simulink model "svc_go_c"  (R2018a)
settings: Solver=VariableStepAuto  StartTime=0.0  StopTime=10.0  RelTol=1e-3
InitFcn:
  | svc_go_init
values from neighbouring files (symbols this model uses):
  kp = (3*Ld./N/Ts-Rs)/Lq/Iq    [est_model_paras.m]    (also in svc_go_init.m = -0.01944)
  Ld = 0.000891    [est_model_paras.m]    (also in svc_go_init.m = 0.00026)
  Ldr = 0.00026    [svc_go_init.m]
  Lq = 0.000891    [est_model_paras.m]    (also in svc_go_init.m = 0.000636)
  Lqr = 0.00053    [svc_go_init.m]
  phi_r = 0.012    [est_model_paras.m]    (also in svc_go_init.m = 0.078)
  Rs = 0.503    [est_model_paras.m]    (also in svc_go_init.m = 0.021)
  Rsr = 0.021    [svc_go_init.m]
  We = 2*pi*100    (= 628.318530718)    [est_model_paras.m]    (also in svc_go_init.m)
libraries: simulink x5
settings Model: Creator=LG-PC  LastModifiedBy=LG-PC

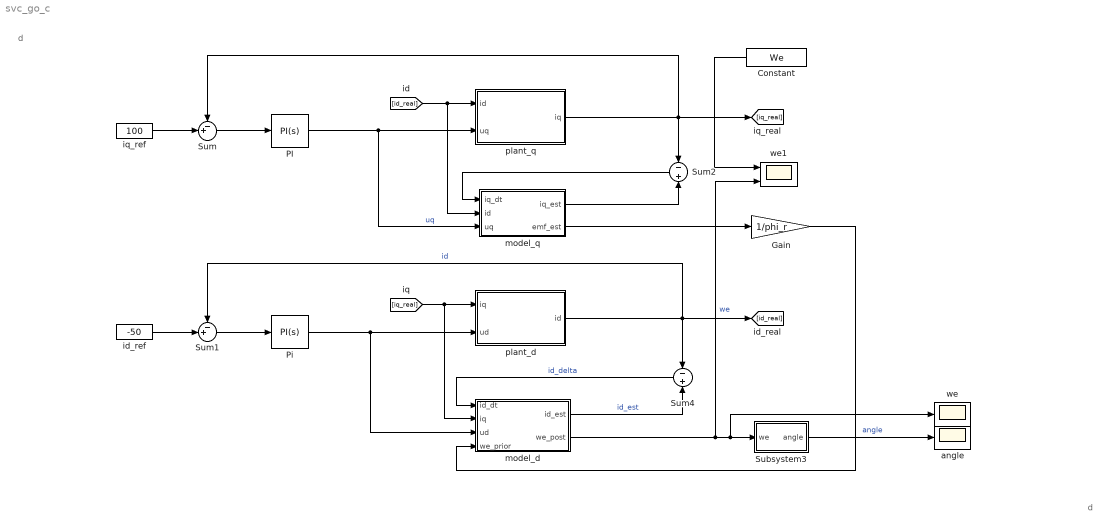
== system svc_go_c ==
  note: d
  note: d
  Constant : Constant  Value=We
  Gain : Gain  Gain=1/phi_r
  PI : simulink/Continuous/PID Controller  Controller=PI  TimeDomain=Continuous-time  SampleTime=-1  IntegratorMethod=Forward Euler  FilterMethod=Forward Euler  Form=Parallel  UseFilter=on  ControllerParametersSource=internal  P=1  I=50  D=0  N=100  InitialConditionSource=internal  InitialConditionForIntegrator=0  InitialConditionForFilter=0  ExternalReset=none  LimitOutput=off  UpperSaturationLimit=inf  LowerSaturationLimit=-inf  LinearizeAsGain=on  AntiWindupMode=none  Kb=1  TrackingMode=off  Kt=1  PParamMin=[]  PParamMax=[]  IParamMin=[]  IParamMax=[]  DParamMin=[]  DParamMax=[]  NParamMin=[]  NParamMax=[]  KbParamMin=[]  KbParamMax=[]  KtParamMin=[]  KtParamMax=[]  POutMin=[]  POutMax=[]  IOutMin=[]  IOutMax=[]  DOutMin=[]  DOutMax=[]  NOutMin=[]  NOutMax=[]  KbOutMin=[]  KbOutMax=[]  KtOutMin=[]  KtOutMax=[]  IntegratorOutMin=[]  IntegratorOutMax=[]  FilterOutMin=[]  FilterOutMax=[]  SumOutMin=[]  SumOutMax=[]  SumI1OutMin=[]  SumI1OutMax=[]  SumI2OutMin=[]  SumI2OutMax=[]  SumI3OutMin=[]  SumI3OutMax=[]  SumDOutMin=[]  SumDOutMax=[]  SaturationOutMin=[]  SaturationOutMax=[]  IntegratorContinuousStateAttributes=''  IntegratorStateMustResolveToSignalObject=off  IntegratorRTWStateStorageClass=Auto  FilterContinuousStateAttributes=''  FilterStateMustResolveToSignalObject=off  FilterRTWStateStorageClass=Auto  DifferentiatorICPrevScaledInput=0  DifferentiatorOutMin=[]  DifferentiatorOutMax=[]  FilterDiffOutCoefMin=[]  FilterDiffOutCoefMax=[]  SumDenOutMin=[]  SumDenOutMax=[]  SumNumOutMin=[]  SumNumOutMax=[]  ReciprocalOutMin=[]  ReciprocalOutMax=[]  DivideOutMin=[]  DivideOutMax=[]  TunerSelectOption=Transfer Function Based (PID Tuner App)
  Pi : simulink/Continuous/PID Controller  Controller=PI  TimeDomain=Continuous-time  SampleTime=-1  IntegratorMethod=Forward Euler  FilterMethod=Forward Euler  Form=Parallel  UseFilter=on  ControllerParametersSource=internal  P=1  I=50  D=0  N=100  InitialConditionSource=internal  InitialConditionForIntegrator=0  InitialConditionForFilter=0  ExternalReset=none  LimitOutput=off  UpperSaturationLimit=inf  LowerSaturationLimit=-inf  LinearizeAsGain=on  AntiWindupMode=none  Kb=1  TrackingMode=off  Kt=1  PParamMin=[]  PParamMax=[]  IParamMin=[]  IParamMax=[]  DParamMin=[]  DParamMax=[]  NParamMin=[]  NParamMax=[]  KbParamMin=[]  KbParamMax=[]  KtParamMin=[]  KtParamMax=[]  POutMin=[]  POutMax=[]  IOutMin=[]  IOutMax=[]  DOutMin=[]  DOutMax=[]  NOutMin=[]  NOutMax=[]  KbOutMin=[]  KbOutMax=[]  KtOutMin=[]  KtOutMax=[]  IntegratorOutMin=[]  IntegratorOutMax=[]  FilterOutMin=[]  FilterOutMax=[]  SumOutMin=[]  SumOutMax=[]  SumI1OutMin=[]  SumI1OutMax=[]  SumI2OutMin=[]  SumI2OutMax=[]  SumI3OutMin=[]  SumI3OutMax=[]  SumDOutMin=[]  SumDOutMax=[]  SaturationOutMin=[]  SaturationOutMax=[]  IntegratorContinuousStateAttributes=''  IntegratorStateMustResolveToSignalObject=off  IntegratorRTWStateStorageClass=Auto  FilterContinuousStateAttributes=''  FilterStateMustResolveToSignalObject=off  FilterRTWStateStorageClass=Auto  DifferentiatorICPrevScaledInput=0  DifferentiatorOutMin=[]  DifferentiatorOutMax=[]  FilterDiffOutCoefMin=[]  FilterDiffOutCoefMax=[]  SumDenOutMin=[]  SumDenOutMax=[]  SumNumOutMin=[]  SumNumOutMax=[]  ReciprocalOutMin=[]  ReciprocalOutMax=[]  DivideOutMin=[]  DivideOutMax=[]  TunerSelectOption=Transfer Function Based (PID Tuner App)
  Subsystem3 : Subsystem
  Sum : Sum  Inputs=-+|
  Sum1 : Sum  Inputs=-+|
  Sum2 : Sum  Inputs=-+
  Sum4 : Sum  Inputs=-+
  angle : Scope
  id_ref : Constant  Value=-50
  iq_ref : Constant  Value=100
  model_d : Subsystem
  model_q : Subsystem
  plant_d : Subsystem
  plant_q : Subsystem
  we : Scope
  we1 : Scope  NumInputPorts=2
  wires:
  PI/1 -> plant_q/2(uq), model_q/3(uq)  "uq"
  Sum/1 -> PI/1
  Sum2/1 -> model_q/1(iq_dt)
  model_q/1(iq_est) -> Sum2/2
  plant_q/1(iq) -> Sum/1, [iq_real], Sum2/1
  [id_real] -> model_q/2(id), plant_q/1(id)
  iq_ref/1 -> Sum/2
  id_ref/1 -> Sum1/2
  Sum1/1 -> Pi/1
  Pi/1 -> model_d/3(ud), plant_d/2(ud)
  plant_d/1(id) -> Sum1/1, Sum4/1, [id_real]  "id"
  [iq_real] -> plant_d/1(iq), model_d/2(iq)
  Sum4/1 -> model_d/1(id_dt)  "id_delta"
  model_d/1(id_est) -> Sum4/2  "id_est"
  Gain/1 -> model_d/4(we_prior)
  model_q/2(emf_est) -> Gain/1
  model_d/2(we_post) -> we1/2, we/1, Subsystem3/1(we)  "we"
  Subsystem3/1(angle) -> angle/1  "angle"
  Constant/1 -> we1/1

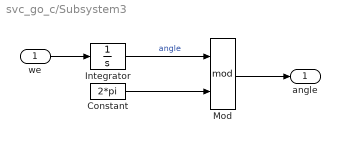
== system svc_go_c/Subsystem3 ==
  we : Inport
  Constant : Constant  Value=2*pi
  Integrator : Integrator
  Mod : Math  Operator=mod  SaturateOnIntegerOverflow=on
  angle : Outport
  wires:
  Constant/1 -> Mod/2
  Integrator/1 -> Mod/1  "angle"
  we/1 -> Integrator/1
  Mod/1 -> angle/1

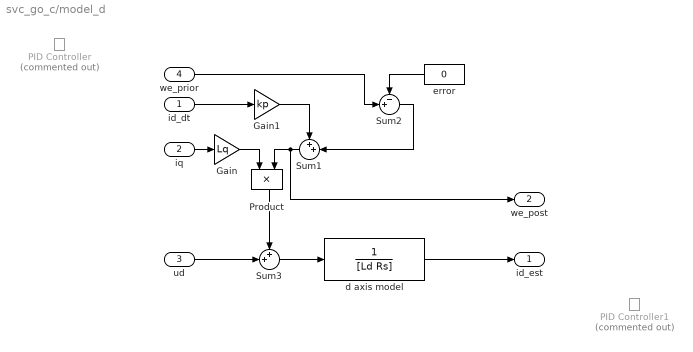
== system svc_go_c/model_d ==
  id_dt : Inport
  iq : Inport  Port=2
  ud : Inport  Port=3
  we_prior : Inport  Port=4
  Gain : Gain  Gain=Lq
  Gain1 : Gain  Gain=kp
  PID Controller : simulink/Continuous/PID Controller  Commented=on  Controller=PI  TimeDomain=Continuous-time  SampleTime=-1  IntegratorMethod=Forward Euler  FilterMethod=Forward Euler  Form=Parallel  UseFilter=on  ControllerParametersSource=internal  P=100  I=0  D=0  N=100  InitialConditionSource=internal  InitialConditionForIntegrator=0  InitialConditionForFilter=0  ExternalReset=none  LimitOutput=off  UpperSaturationLimit=inf  LowerSaturationLimit=-inf  LinearizeAsGain=on  AntiWindupMode=none  Kb=1  TrackingMode=off  Kt=1  PParamMin=[]  PParamMax=[]  IParamMin=[]  IParamMax=[]  DParamMin=[]  DParamMax=[]  NParamMin=[]  NParamMax=[]  KbParamMin=[]  KbParamMax=[]  KtParamMin=[]  KtParamMax=[]  POutMin=[]  POutMax=[]  IOutMin=[]  IOutMax=[]  DOutMin=[]  DOutMax=[]  NOutMin=[]  NOutMax=[]  KbOutMin=[]  KbOutMax=[]  KtOutMin=[]  KtOutMax=[]  IntegratorOutMin=[]  IntegratorOutMax=[]  FilterOutMin=[]  FilterOutMax=[]  SumOutMin=[]  SumOutMax=[]  SumI1OutMin=[]  SumI1OutMax=[]  SumI2OutMin=[]  SumI2OutMax=[]  SumI3OutMin=[]  SumI3OutMax=[]  SumDOutMin=[]  SumDOutMax=[]  SaturationOutMin=[]  SaturationOutMax=[]  IntegratorContinuousStateAttributes=''  IntegratorStateMustResolveToSignalObject=off  IntegratorRTWStateStorageClass=Auto  FilterContinuousStateAttributes=''  FilterStateMustResolveToSignalObject=off  FilterRTWStateStorageClass=Auto  DifferentiatorICPrevScaledInput=0  DifferentiatorOutMin=[]  DifferentiatorOutMax=[]  FilterDiffOutCoefMin=[]  FilterDiffOutCoefMax=[]  SumDenOutMin=[]  SumDenOutMax=[]  SumNumOutMin=[]  SumNumOutMax=[]  ReciprocalOutMin=[]  ReciprocalOutMax=[]  DivideOutMin=[]  DivideOutMax=[]  TunerSelectOption=Transfer Function Based (PID Tuner App)
  PID Controller1 : simulink/Continuous/PID Controller  Commented=on  Controller=PI  TimeDomain=Continuous-time  SampleTime=-1  IntegratorMethod=Forward Euler  FilterMethod=Forward Euler  Form=Parallel  UseFilter=on  ControllerParametersSource=internal  P=100  I=0  D=0  N=100  InitialConditionSource=internal  InitialConditionForIntegrator=0  InitialConditionForFilter=0  ExternalReset=none  LimitOutput=off  UpperSaturationLimit=inf  LowerSaturationLimit=-inf  LinearizeAsGain=on  AntiWindupMode=none  Kb=1  TrackingMode=off  Kt=1  PParamMin=[]  PParamMax=[]  IParamMin=[]  IParamMax=[]  DParamMin=[]  DParamMax=[]  NParamMin=[]  NParamMax=[]  KbParamMin=[]  KbParamMax=[]  KtParamMin=[]  KtParamMax=[]  POutMin=[]  POutMax=[]  IOutMin=[]  IOutMax=[]  DOutMin=[]  DOutMax=[]  NOutMin=[]  NOutMax=[]  KbOutMin=[]  KbOutMax=[]  KtOutMin=[]  KtOutMax=[]  IntegratorOutMin=[]  IntegratorOutMax=[]  FilterOutMin=[]  FilterOutMax=[]  SumOutMin=[]  SumOutMax=[]  SumI1OutMin=[]  SumI1OutMax=[]  SumI2OutMin=[]  SumI2OutMax=[]  SumI3OutMin=[]  SumI3OutMax=[]  SumDOutMin=[]  SumDOutMax=[]  SaturationOutMin=[]  SaturationOutMax=[]  IntegratorContinuousStateAttributes=''  IntegratorStateMustResolveToSignalObject=off  IntegratorRTWStateStorageClass=Auto  FilterContinuousStateAttributes=''  FilterStateMustResolveToSignalObject=off  FilterRTWStateStorageClass=Auto  DifferentiatorICPrevScaledInput=0  DifferentiatorOutMin=[]  DifferentiatorOutMax=[]  FilterDiffOutCoefMin=[]  FilterDiffOutCoefMax=[]  SumDenOutMin=[]  SumDenOutMax=[]  SumNumOutMin=[]  SumNumOutMax=[]  ReciprocalOutMin=[]  ReciprocalOutMax=[]  DivideOutMin=[]  DivideOutMax=[]  TunerSelectOption=Transfer Function Based (PID Tuner App)
  Product : Product
  Sum1 : Sum  Inputs=++|
  Sum2 : Sum  Inputs=-+|
  Sum3 : Sum  Inputs=++|
  d axis model : TransferFcn  Denominator=[Ld Rs]
  error : Constant  Value=0
  id_est : Outport
  we_post : Outport  Port=2
  wires:
  Sum3/1 -> d axis model/1
  iq/1 -> Gain/1
  ud/1 -> Sum3/2
  d axis model/1 -> id_est/1
  Gain/1 -> Product/1
  Product/1 -> Sum3/1
  Sum1/1 -> we_post/1, Product/2
  id_dt/1 -> Gain1/1
  we_prior/1 -> Sum2/2
  Gain1/1 -> Sum1/1
  error/1 -> Sum2/1
  Sum2/1 -> Sum1/2

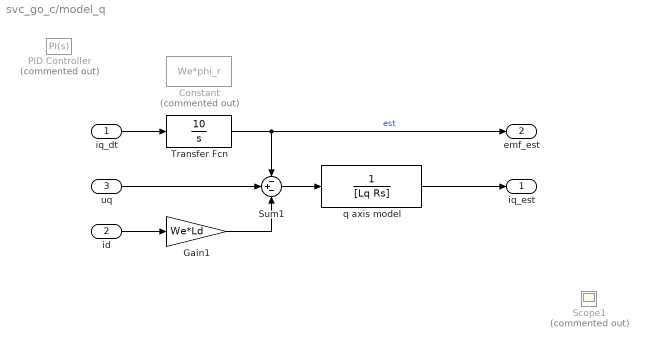
== system svc_go_c/model_q ==
  iq_dt : Inport
  id : Inport  Port=2
  uq : Inport  Port=3
  Constant : Constant  Commented=on  Value=We*phi_r
  Gain1 : Gain  Gain=We*Ld
  PID Controller : simulink/Continuous/PID Controller  Commented=on  Controller=PI  TimeDomain=Continuous-time  SampleTime=-1  IntegratorMethod=Forward Euler  FilterMethod=Forward Euler  Form=Parallel  UseFilter=on  ControllerParametersSource=internal  P=0  I=1.2  D=0  N=100  InitialConditionSource=internal  InitialConditionForIntegrator=0  InitialConditionForFilter=0  ExternalReset=none  LimitOutput=off  UpperSaturationLimit=inf  LowerSaturationLimit=-inf  LinearizeAsGain=on  AntiWindupMode=none  Kb=1  TrackingMode=off  Kt=1  PParamMin=[]  PParamMax=[]  IParamMin=[]  IParamMax=[]  DParamMin=[]  DParamMax=[]  NParamMin=[]  NParamMax=[]  KbParamMin=[]  KbParamMax=[]  KtParamMin=[]  KtParamMax=[]  POutMin=[]  POutMax=[]  IOutMin=[]  IOutMax=[]  DOutMin=[]  DOutMax=[]  NOutMin=[]  NOutMax=[]  KbOutMin=[]  KbOutMax=[]  KtOutMin=[]  KtOutMax=[]  IntegratorOutMin=[]  IntegratorOutMax=[]  FilterOutMin=[]  FilterOutMax=[]  SumOutMin=[]  SumOutMax=[]  SumI1OutMin=[]  SumI1OutMax=[]  SumI2OutMin=[]  SumI2OutMax=[]  SumI3OutMin=[]  SumI3OutMax=[]  SumDOutMin=[]  SumDOutMax=[]  SaturationOutMin=[]  SaturationOutMax=[]  IntegratorContinuousStateAttributes=''  IntegratorStateMustResolveToSignalObject=off  IntegratorRTWStateStorageClass=Auto  FilterContinuousStateAttributes=''  FilterStateMustResolveToSignalObject=off  FilterRTWStateStorageClass=Auto  DifferentiatorICPrevScaledInput=0  DifferentiatorOutMin=[]  DifferentiatorOutMax=[]  FilterDiffOutCoefMin=[]  FilterDiffOutCoefMax=[]  SumDenOutMin=[]  SumDenOutMax=[]  SumNumOutMin=[]  SumNumOutMax=[]  ReciprocalOutMin=[]  ReciprocalOutMax=[]  DivideOutMin=[]  DivideOutMax=[]  TunerSelectOption=Transfer Function Based (PID Tuner App)
  Scope1 : Scope  Commented=on  NumInputPorts=2
  Sum1 : Sum  Inputs=-+-
  Transfer Fcn : TransferFcn  Numerator=[10]  Denominator=[1 0]
  q axis model : TransferFcn  Denominator=[Lq Rs]
  iq_est : Outport
  emf_est : Outport  Port=2
  wires:
  id/1 -> Gain1/1
  Gain1/1 -> Sum1/3
  q axis model/1 -> iq_est/1
  iq_dt/1 -> Transfer Fcn/1
  Sum1/1 -> q axis model/1
  uq/1 -> Sum1/2
  Transfer Fcn/1 -> Sum1/1, emf_est/1  "est"

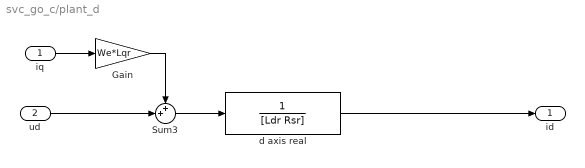
== system svc_go_c/plant_d ==
  iq : Inport
  ud : Inport  Port=2
  Gain : Gain  Gain=We*Lqr
  Sum3 : Sum  Inputs=++|
  d axis real : TransferFcn  Denominator=[Ldr Rsr]
  id : Outport
  wires:
  Sum3/1 -> d axis real/1
  iq/1 -> Gain/1
  ud/1 -> Sum3/2
  d axis real/1 -> id/1
  Gain/1 -> Sum3/1

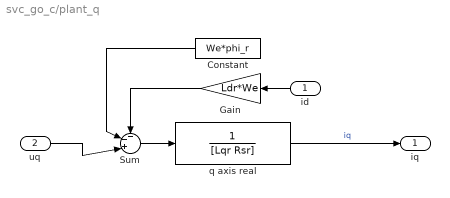
== system svc_go_c/plant_q ==
  id : Inport
  uq : Inport  Port=2
  Constant : Constant  Value=We*phi_r
  Gain : Gain  Gain=Ldr*We
  Sum : Sum  Inputs=--+|
  q axis real : TransferFcn  Denominator=[Lqr Rsr]
  iq : Outport
  wires:
  id/1 -> Gain/1
  q axis real/1 -> iq/1  "iq"
  Sum/1 -> q axis real/1
  uq/1 -> Sum/3
  Gain/1 -> Sum/1
  Constant/1 -> Sum/2
